simulink model "project_2023_12_4_P71"  (R2017b)
settings: Solver=VariableStepAuto  StartTime=0.0  StopTime=100  RelTol=1e-3
settings Model: Creator=Administrator  LastModifiedBy=Administrator

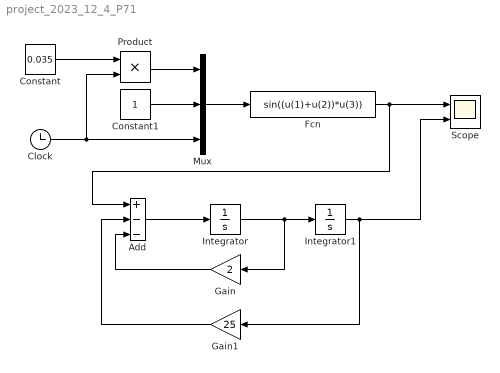
== system project_2023_12_4_P71 ==
  Add : Sum  Inputs=+--
  Clock : Clock
  Constant : Constant  Value=0.035
  Constant1 : Constant
  Fcn : Fcn  Expr=sin((u(1)+u(2))*u(3))
  Gain : Gain  Gain=2
  Gain1 : Gain  Gain=25
  Integrator : Integrator
  Integrator1 : Integrator
  Mux : Mux  Inputs=3
  Product : Product
  Scope : Scope  NumInputPorts=2
  wires:
  Constant/1 -> Product/1
  Product/1 -> Mux/1
  Constant1/1 -> Mux/2
  Clock/1 -> Product/2, Mux/3
  Mux/1 -> Fcn/1
  Fcn/1 -> Add/1, Scope/1
  Add/1 -> Integrator/1
  Integrator/1 -> Gain/1, Integrator1/1
  Gain/1 -> Add/3
  Integrator1/1 -> Scope/2, Gain1/1
  Gain1/1 -> Add/2
